simulink model "test_ESI_power_design"  (Simulink 4.00)
settings: Solver=FixedStepDiscrete  StartTime=0.0  StopTime=100  FixedStep=parameters.model.sample_time  RelTol=1e-3
undefined symbols (not defined in the file or in its folder): parameters
libraries: controller_design_lib x1, IdInput_block_lib x1, save_blocks_lib x1
settings Model: LastModifiedBy=bsaunder

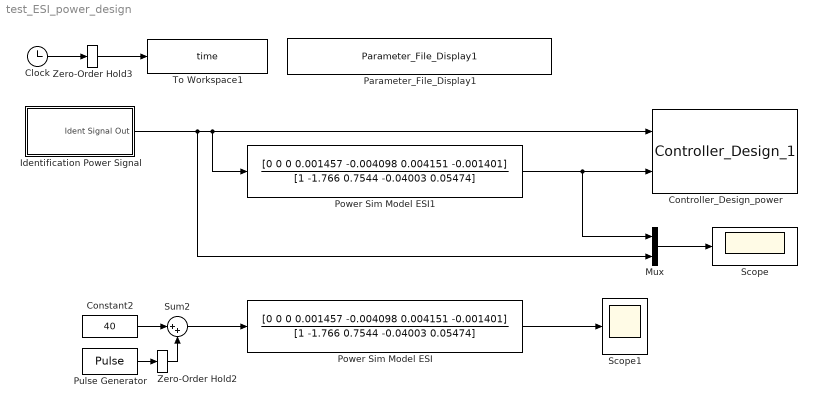
== system test_ESI_power_design ==
  Clock : Clock
      settings: DisplayTime=off  Decimation=10
  Constant2 : Constant  Value=40
  Controller_Design_power : controller_design_lib/Controller_Design_1  cntr_orders=parameters.power_control_design.orders  ctrObs_dyn=parameters.power_control_design.control_observer_dynamics  refMdl_dyn=parameters.power_control_design.reference_model_dynamics  Ts=parameters.power_controller.sample_time
  Identification Power Signal : Subsystem
      settings: RTWFcnNameOpts=Auto  RTWFileNameOpts=Auto
  Mux : Mux  Inputs=2
  Parameter_File_Display1 : save_blocks_lib/Parameter_File_Display1
  Power Sim Model ESI : DiscreteFilter  Numerator=[0 0 0 0.001457 -0.004098 0.004151 -0.001401]  Denominator=[1 -1.766 0.7544 -0.04003 0.05474]  SampleTime=0.05  Realization=auto
      settings: RTWStateStorageClass=Auto
  Power Sim Model ESI1 : DiscreteFilter  Numerator=[0 0 0 0.001457 -0.004098 0.004151 -0.001401]  Denominator=[1 -1.766 0.7544 -0.04003 0.05474]  SampleTime=0.05  Realization=auto
      settings: RTWStateStorageClass=Auto
  Pulse Generator : DiscretePulseGenerator  PulseType=Time-based  Amplitude=20  Period=40  PulseWidth=50  PhaseDelay=0  SampleTime=1
  Scope : Scope
      settings: TimeRange=auto  YMin=0  YMax=120  SaveToWorkspace=off  SaveName=ScopeData  LimitDataPoints=on  MaxDataPoints=5000
  Scope1 : Scope
      settings: TimeRange=60  YMin=0  YMax=70  SaveToWorkspace=off  LimitDataPoints=on  MaxDataPoints=5000
  Sum2 : Sum  Inputs=|++  SaturateOnIntegerOverflow=on
  To Workspace1 : ToWorkspace  VariableName=time  SampleTime=parameters.sample_time  SaveFormat=Array
  Zero-Order Hold2 : ZeroOrderHold  SampleTime=parameters.sample_time
  Zero-Order Hold3 : ZeroOrderHold  SampleTime=parameters.sample_time
  wires:
  Mux/1 -> Scope/1
  Clock/1 -> Zero-Order Hold3/1
  Constant2/1 -> Sum2/1
  Pulse Generator/1 -> Zero-Order Hold2/1
  Sum2/1 -> Power Sim Model ESI/1
  Power Sim Model ESI/1 -> Scope1/1
  Power Sim Model ESI1/1 -> Mux/1, Controller_Design_power/2
  Identification Power Signal/1(Ident Signal Out) -> Controller_Design_power/1, Power Sim Model ESI1/1, Mux/2
  Zero-Order Hold2/1 -> Sum2/2
  Zero-Order Hold3/1 -> To Workspace1/1

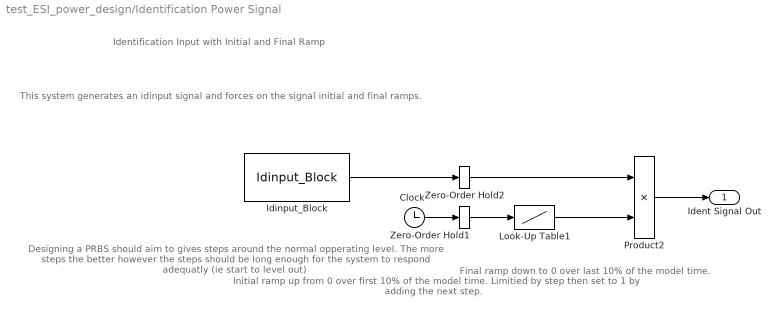
== system test_ESI_power_design/Identification Power Signal ==
  note: Initial ramp up from 0 over
      | first 10% of the model time.
      | Limitied by step then set to
      | 1 by adding the next step.
  note: Final ramp down to 0 over last
      | 10% of the model time.
  note: This system generates an
      | idinput signal and forces on
      | the signal initial and final
      | ramps.
  note: Identification Input with Initial and Final Ramp
  note: Designing a PRBS should aim
      | to gives steps around the normal
      | opperating level.  The more
      | steps the better however the
      | steps should be long enough for
      | the system to respond adequatly
      | (ie start to level out)
  Clock : Clock
      settings: DisplayTime=off  Decimation=10
  Idinput_Block : IdInput_block_lib/Idinput_Block  ssT=[0.1*parameters.power_identification.total_time 0.9*parameters.power_identification.total_time]  signal_type=PRBS  band=[0 1/parameters.power_PRBS.min_same_time]  levels=parameters.power_PRBS.output_limits  Ts=parameters.sample_time
  Look-Up Table1 : Lookup  InputValues=[0 0.1 0.9 1.0].*parameters.power_identification.total_time  OutputValues=[0 1 1 0]
  Product2 : Product  Inputs=2  Multiplication=Element-wise(.*)  SaturateOnIntegerOverflow=on
  Zero-Order Hold1 : ZeroOrderHold  SampleTime=parameters.sample_time
  Zero-Order Hold2 : ZeroOrderHold  SampleTime=parameters.sample_time
  Ident Signal Out : Outport  Port=1
  wires:
  Product2/1 -> Ident Signal Out/1
  Idinput_Block/1 -> Zero-Order Hold2/1
  Zero-Order Hold2/1 -> Product2/1
  Clock/1 -> Zero-Order Hold1/1
  Look-Up Table1/1 -> Product2/2
  Zero-Order Hold1/1 -> Look-Up Table1/1
